simulink model "pid_sys_sf"  (R2017b)
settings: Solver=VariableStepAuto  StartTime=0.0  StopTime=100  RelTol=1e-3
libraries: simulink_extras x4, simulink x2
settings Model: Creator=Iman  LastModifiedBy=Iman

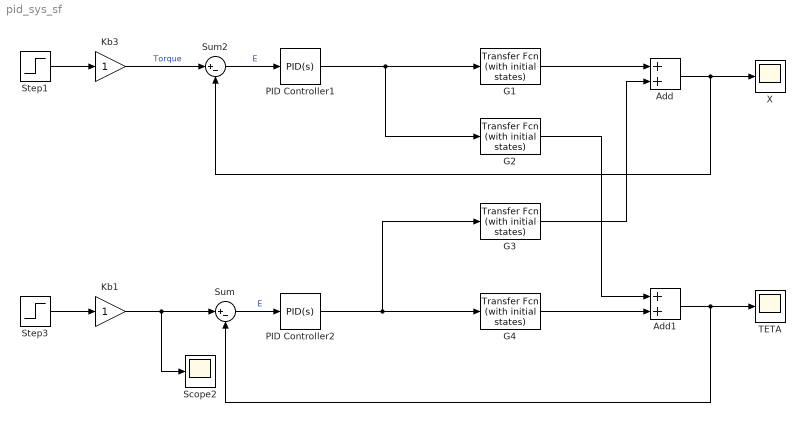
== system pid_sys_sf ==
  Add : Sum
  Add1 : Sum
  G1 : simulink_extras/Additional Linear/Transfer Fcn (with initial states)  N=[104.5 -2150 -3.368e04 -6.03e04]  D=[1 2564 3.781e04 1.506e05 7.832e04 0]  X0=0
  G2 : simulink_extras/Additional Linear/Transfer Fcn (with initial states)  N=[-1374 -8.86e04 -6.695e05]  D=[1 2564 3.781e04 1.506e05 7.832e04]  X0=0
  G3 : simulink_extras/Additional Linear/Transfer Fcn (with initial states)  N=[104.5 -2506 -2.32e04 -3.682e04]  D=[1 2564 3.781e04 1.506e05 7.832e04 0]  X0=0
  G4 : simulink_extras/Additional Linear/Transfer Fcn (with initial states)  N=[-1374 -8.393e04 -4.088e05]  D=[1 2564 3.781e04 1.506e05 7.832e04]  X0=0
  Kb1 : Gain
  Kb3 : Gain
  PID Controller1 : simulink/Continuous/PID Controller  Controller=PID  TimeDomain=Continuous-time  SampleTime=-1  IntegratorMethod=Forward Euler  FilterMethod=Forward Euler  Form=Parallel  UseFilter=on  ControllerParametersSource=internal  P=-2.36034954173394  I=-0.483360554643987  D=-2.0198788764389  N=2.04805786678134  InitialConditionSource=internal  InitialConditionForIntegrator=0  InitialConditionForFilter=0  ExternalReset=none  LimitOutput=off  UpperSaturationLimit=inf  LowerSaturationLimit=-inf  LinearizeAsGain=on  AntiWindupMode=none  Kb=1  TrackingMode=off  Kt=1  PParamMin=[]  PParamMax=[]  IParamMin=[]  IParamMax=[]  DParamMin=[]  DParamMax=[]  NParamMin=[]  NParamMax=[]  KbParamMin=[]  KbParamMax=[]  KtParamMin=[]  KtParamMax=[]  POutMin=[]  POutMax=[]  IOutMin=[]  IOutMax=[]  DOutMin=[]  DOutMax=[]  NOutMin=[]  NOutMax=[]  KbOutMin=[]  KbOutMax=[]  KtOutMin=[]  KtOutMax=[]  IntegratorOutMin=[]  IntegratorOutMax=[]  FilterOutMin=[]  FilterOutMax=[]  SumOutMin=[]  SumOutMax=[]  SumI1OutMin=[]  SumI1OutMax=[]  SumI2OutMin=[]  SumI2OutMax=[]  SumI3OutMin=[]  SumI3OutMax=[]  SumDOutMin=[]  SumDOutMax=[]  SaturationOutMin=[]  SaturationOutMax=[]  IntegratorContinuousStateAttributes=''  IntegratorStateMustResolveToSignalObject=off  IntegratorRTWStateStorageClass=Auto  FilterContinuousStateAttributes=''  FilterStateMustResolveToSignalObject=off  FilterRTWStateStorageClass=Auto  DifferentiatorICPrevScaledInput=0  DifferentiatorOutMin=[]  DifferentiatorOutMax=[]  InitialConditionSetting=State (most efficient)  FilterDiffOutCoefMin=[]  FilterDiffOutCoefMax=[]  SumDenOutMin=[]  SumDenOutMax=[]  SumNumOutMin=[]  SumNumOutMax=[]  ReciprocalOutMin=[]  ReciprocalOutMax=[]  DivideOutMin=[]  DivideOutMax=[]  TunerSelectOption=Transfer Function Based (PID Tuner App)
  PID Controller2 : simulink/Continuous/PID Controller  Controller=PID  TimeDomain=Continuous-time  SampleTime=-1  IntegratorMethod=Forward Euler  FilterMethod=Forward Euler  Form=Parallel  UseFilter=on  ControllerParametersSource=internal  P=-5.514003493081  I=-11.313186617116  D=-0.224032526959822  N=129.502250487668  InitialConditionSource=internal  InitialConditionForIntegrator=0  InitialConditionForFilter=0  ExternalReset=none  LimitOutput=off  UpperSaturationLimit=inf  LowerSaturationLimit=-inf  LinearizeAsGain=on  AntiWindupMode=none  Kb=1  TrackingMode=off  Kt=1  PParamMin=[]  PParamMax=[]  IParamMin=[]  IParamMax=[]  DParamMin=[]  DParamMax=[]  NParamMin=[]  NParamMax=[]  KbParamMin=[]  KbParamMax=[]  KtParamMin=[]  KtParamMax=[]  POutMin=[]  POutMax=[]  IOutMin=[]  IOutMax=[]  DOutMin=[]  DOutMax=[]  NOutMin=[]  NOutMax=[]  KbOutMin=[]  KbOutMax=[]  KtOutMin=[]  KtOutMax=[]  IntegratorOutMin=[]  IntegratorOutMax=[]  FilterOutMin=[]  FilterOutMax=[]  SumOutMin=[]  SumOutMax=[]  SumI1OutMin=[]  SumI1OutMax=[]  SumI2OutMin=[]  SumI2OutMax=[]  SumI3OutMin=[]  SumI3OutMax=[]  SumDOutMin=[]  SumDOutMax=[]  SaturationOutMin=[]  SaturationOutMax=[]  IntegratorContinuousStateAttributes=''  IntegratorStateMustResolveToSignalObject=off  IntegratorRTWStateStorageClass=Auto  FilterContinuousStateAttributes=''  FilterStateMustResolveToSignalObject=off  FilterRTWStateStorageClass=Auto  DifferentiatorICPrevScaledInput=0  DifferentiatorOutMin=[]  DifferentiatorOutMax=[]  InitialConditionSetting=State (most efficient)  FilterDiffOutCoefMin=[]  FilterDiffOutCoefMax=[]  SumDenOutMin=[]  SumDenOutMax=[]  SumNumOutMin=[]  SumNumOutMax=[]  ReciprocalOutMin=[]  ReciprocalOutMax=[]  DivideOutMin=[]  DivideOutMax=[]  TunerSelectOption=Transfer Function Based (PID Tuner App)
  Scope2 : Scope
  Step1 : Step  Time=0  SampleTime=0.1
  Step3 : Step  Time=0  SampleTime=0.1
  Sum : Sum  Inputs=|+-
  Sum2 : Sum  Inputs=|+-
  TETA : Scope
  X : Scope
  wires:
  PID Controller1/1 -> G2/1, G1/1
  G4/1 -> Add1/2
  G1/1 -> Add/1
  G3/1 -> Add/2
  G2/1 -> Add1/1
  Add/1 -> Sum2/2, X/1
  Step1/1 -> Kb3/1
  Step3/1 -> Kb1/1
  Sum/1 -> PID Controller2/1  "E"
  Kb3/1 -> Sum2/1  "Torque"
  Kb1/1 -> Scope2/1, Sum/1
  Sum2/1 -> PID Controller1/1  "E"
  Add1/1 -> Sum/2, TETA/1
  PID Controller2/1 -> G3/1, G4/1
